simulink subsystem "Regular_Operation"  (R2023b)
settings: Solver=VariableStepAuto  StartTime=0.0  StopTime=10.0  RelTol=1e-3
settings Model: Creator=nickj  LastModifiedBy=heyka

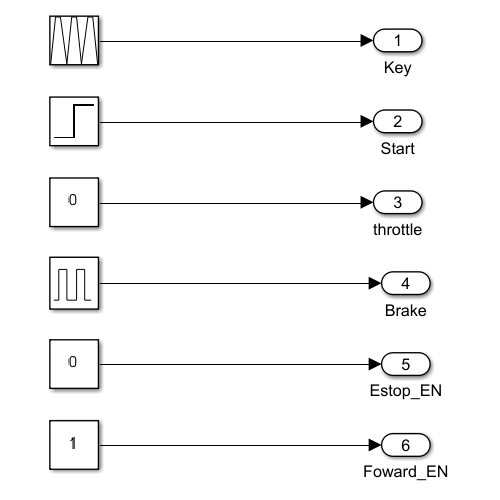
[thumbnail: Simulink's stored preview of the top-level diagram]
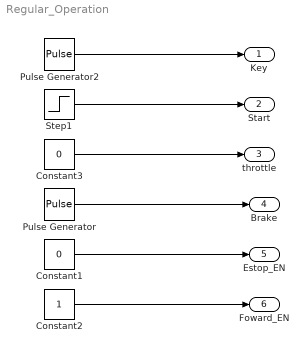
== system Regular_Operation ==
  Constant1 : Constant  Value=0
  Constant2 : Constant
  Constant3 : Constant  Value=0
  Pulse Generator : DiscretePulseGenerator  Period=500  PulseWidth=300  PhaseDelay=200
  Pulse Generator2 : DiscretePulseGenerator  Period=500  PulseWidth=300  PhaseDelay=100
  Step1 : Step  Time=200  SampleTime=0
  Key : Outport
  Start : Outport  Port=2
  throttle : Outport  Port=3
  Brake : Outport  Port=4
  Estop_EN : Outport  Port=5
  Foward_EN : Outport  Port=6
  wires:
  Constant1/1 -> Estop_EN/1
  Constant2/1 -> Foward_EN/1
  Constant3/1 -> throttle/1
  Step1/1 -> Start/1
  Pulse Generator2/1 -> Key/1
  Pulse Generator/1 -> Brake/1
